simulink library "Prop_demo"  (R2025b)
settings: Solver=VariableStepAuto  StartTime=0.0  StopTime=10.0  RelTol=1e-3
undefined symbols (not defined in the file): cfd2d_ja, cfd2d_jl, cfd2d_kQ, cfd2d_kT, cfd2d_P1_CEF_X, cfd2d_P1_CEF_Y, cfd2d_P1_CEF_Z, cfd2d_P1_CEM_X, cfd2d_P1_CEM_Y, cfd2d_P1_CEM_Z, cfd2d_P5_CEF_X, cfd2d_P5_CEF_Y, cfd2d_P5_CEF_Z, cfd2d_P5_CEM_X, cfd2d_P5_CEM_Y, cfd2d_P5_CEM_Z, cfd3d_ja, cfd3d_jl, cfd3d_P2_CEF_X, cfd3d_P2_CEF_Y, cfd3d_P2_CEF_Z, cfd3d_P2_CEM_X, cfd3d_P2_CEM_Y, cfd3d_P2_CEM_Z, cfd3d_P6_CEF_X, cfd3d_P6_CEF_Y, cfd3d_P6_CEF_Z, cfd3d_P6_CEM_X, cfd3d_P6_CEM_Y, cfd3d_P6_CEM_Z, cfd3d_pitch, CoefBus, DF3000_V2_Prop, magnitude, Prop1, Prop2
libraries: simulink_extras x22, matrix_library x12, sharedtransform x12, simulink x6, DF3000_V2_Common x4
(part 1 of 4)
settings Model: Creator=someone  LastModifiedBy=someone

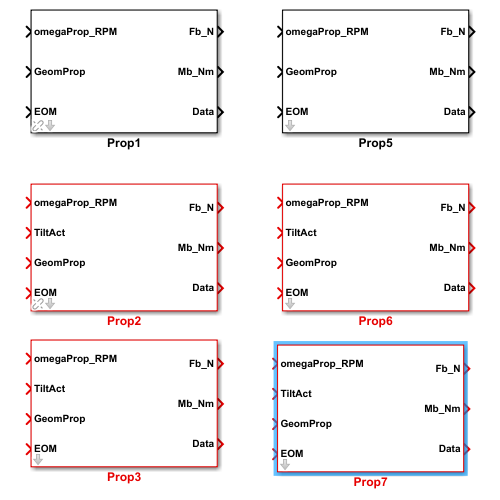
[thumbnail: Simulink's stored preview of the top-level diagram]
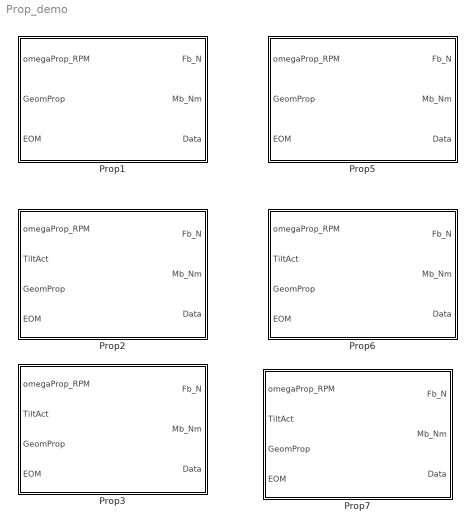
== system Prop_demo ==
  Prop1 : Subsystem  AncestorBlock=DF3000_V2_Prop/Prop1  mask{propAbs=1}
      mask prompts: propAbs "Prop Index"
      mask DialogControl ParameterGroupVar Prompt: 参数
  Prop2 : Subsystem  AncestorBlock=DF3000_V2_Prop/Prop2  mask{propAbs=2, ArmDirSelected=on}
      mask prompts: propAbs "Prop Index"; ArmDirSelected "Positive Installed (Front Prop)"
      mask DialogControl ParameterGroupVar Prompt: 参数
  Prop3 : Subsystem  mask{propAbs=2, ArmDirSelected=on}
      mask prompts: propAbs "Prop Index"; ArmDirSelected "Positive Installed (Front Prop)"
      mask DialogControl ParameterGroupVar Prompt: 参数
  Prop5 : Subsystem  mask{propAbs=5}
      mask prompts: propAbs "Prop Index"
      mask DialogControl ParameterGroupVar Prompt: 参数
  Prop6 : Subsystem  mask{propAbs=6, ArmDirSelected=on}
      mask prompts: propAbs "Prop Index"; ArmDirSelected "Positive Installed (Front Prop)"
      mask DialogControl ParameterGroupVar Prompt: 参数
  Prop7 : Subsystem  mask{propAbs=6, ArmDirSelected=on}
      mask prompts: propAbs "Prop Index"; ArmDirSelected "Positive Installed (Front Prop)"
      mask DialogControl ParameterGroupVar Prompt: 参数

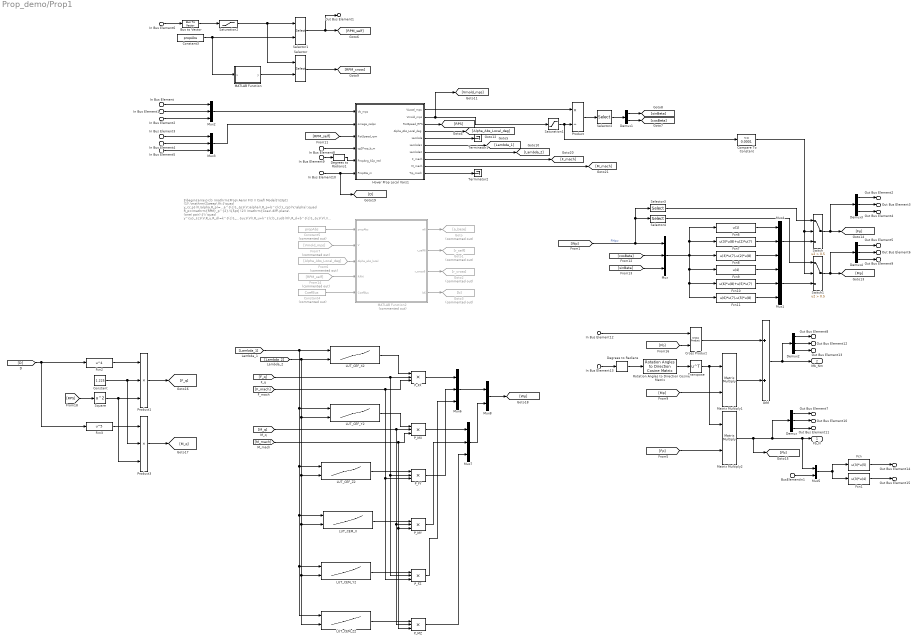
== system Prop_demo/Prop1 ==
  note: $\begin{array}{l} \mathrm{Prop\ Aero\ Fit\ /\ Coef\ Model}\\[3pt] (1)\ \mathrm{Sweep\ fit:}\quad y_{c,p}(V,\alpha,R_p)=a^{(c)}_{p}(V,\alpha)\,R_p+b^{(c)}_{p}(V,\alpha),\quad R_p=\mathrm{RPM}_p^{2}.\\[5pt] (2)\ \mathrm{Coax\ diff\ plane\ (one\ pair):}\\ \quad y^{u}_{c}(V,R_u,R_d)=k^{(c)}_{uu}(V)\,R_u+k^{(c)}_{ud}(V)\,R_d+b^{(c)}_{u}(V),\\ \quad y^{d}_{c}(V,R_u,R_d)=k^{(c)}_{du}(V)\,R_u+k^{(c)}_{dd}(V)\,R_d+b^{(c)}_{d}(V).\\[5pt] (3)\ \mathrm{Ratio\ (split\ of\ slope):}\quad s^{(c)}_{u}=k^{(c)}_{uu}+k^{(c)}_{ud},\quad s^{(c)}_{d}=k^{(c)}_{dd}+k^{(c)}_{du},\\ \quad r^{(c)}_{uu}=\frac{k^{(c)}_{uu}}{s^{(c)}_{u}},\quad r^{(c)}_{ud}=\frac{k^{(c)}_{ud}}{s^{(c)}_{u}},\quad r^{(c)}_{dd}=\frac{k^{(c)}_{dd}}{s^{(c)}_{d}},\quad r^{(c)}_{du}=\frac{k^{(c)}_{du}}{s^{(c)}_{d}}.\\[5pt] (4)\ \mathrm{Coax\ weight:}\quad s=(\cos(\alpha))^{p},\quad p=\mathrm{coaxAlphaPow}.\\ \quad \mathrm{upper:}\quad a^{(c)}_{\mathrm{self}}=s\,r^{(c)}_{uu}\,a^{(c)}_{p},\quad a^{(c)}_{\mathrm{cross}}=s\,r^{(c)}_{ud}\,a^{(c)}_{p},\\ \quad \mathrm{lower:}\quad a^{(c)}_{\mathrm{self}}=s\,r^{(c)}_{dd}\,a^{(c)}_{p},\quad a^{(c)}_{\mathrm{cross}}=s\,r^{(c)}_{du}\,a^{(c)}_{p}.\\[5pt] (5)\ \mathrm{Final\ prediction:}\quad \hat y_{c,p}=a^{(c)}_{\mathrm{self}}\,R_p+a^{(c)}_{\mathrm{cross}}\,R_{m(p)}+b^{(c)}_{p}(V,\alpha). \end{array}$
  In Bus Element6 : Inport  PortName=omegaProp_RPM
      settings: AttributesFormatString=%<OutDataTypeStr>\nDimensions: %<PortDimensions>
  In Bus Element12 : Inport  Port=2  PortName=GeomProp  Element=cg2Prop_b_m
      settings: AttributesFormatString=%<OutDataTypeStr>\nDimensions: %<PortDimensions>
  In Bus Element8 : Inport  Port=2  PortName=GeomProp  Element=cg2Prop_b_m
      settings: AttributesFormatString=%<OutDataTypeStr>\nDimensions: %<PortDimensions>
  In Bus Element13 : Inport  Port=2  PortName=GeomProp  Element=PropAng_b2p_deg
      settings: AttributesFormatString=%<OutDataTypeStr>\nDimensions: %<PortDimensions>
  In Bus Element9 : Inport  Port=2  PortName=GeomProp  Element=PropAng_b2p_deg
      settings: AttributesFormatString=%<OutDataTypeStr>\nDimensions: %<PortDimensions>
  In Bus Element10 : Inport  Port=2  PortName=GeomProp  Element=PropDia_m
      settings: AttributesFormatString=%<OutDataTypeStr>\nDimensions: %<PortDimensions>
  BusElementIn1 : Inport  Port=2  PortName=GeomProp  Element=root2Prop_b_m
  In Bus Element : Inport  Port=3  PortName=EOM  Element=VB_mps.Ub_mps
      settings: AttributesFormatString=%<OutDataTypeStr>\nDimensions: %<PortDimensions>
  In Bus Element1 : Inport  Port=3  PortName=EOM  Element=VB_mps.Vb_mps
      settings: AttributesFormatString=%<OutDataTypeStr>\nDimensions: %<PortDimensions>
  In Bus Element2 : Inport  Port=3  PortName=EOM  Element=VB_mps.Wb_mps
      settings: AttributesFormatString=%<OutDataTypeStr>\nDimensions: %<PortDimensions>
  In Bus Element3 : Inport  Port=3  PortName=EOM  Element=Rates_radps.P_radps
      settings: AttributesFormatString=%<OutDataTypeStr>\nDimensions: %<PortDimensions>
  In Bus Element4 : Inport  Port=3  PortName=EOM  Element=Rates_radps.Q_radps
      settings: AttributesFormatString=%<OutDataTypeStr>\nDimensions: %<PortDimensions>
  In Bus Element5 : Inport  Port=3  PortName=EOM  Element=Rates_radps.R_radps
      settings: AttributesFormatString=%<OutDataTypeStr>\nDimensions: %<PortDimensions>
  Add : Sum
  Bus to Vector : BusToVector
  Compare To Constant : simulink/Logic and Bit Operations/Compare To Constant  relop=<=  const=0.0001  OutDataTypeStr=boolean
  Constant : Constant  Value=1.225
  Constant3 : Constant  Value=propAbs
  Constant4 : Constant  Commented=on  Value=CoefBus  OutDataTypeStr=Bus: CoefBusObj
  Constant5 : Constant  Commented=on  Value=propAbs
  Cross Product : matrix_library/Cross Product
  Degrees to Radians : simulink_extras/Transformations/Degrees to Radians
  Degrees to Radians1 : simulink_extras/Transformations/Degrees to Radians
  Demux{,2..4} (4 alike) : Demux  Outputs=3
  Demux1 : Demux  Outputs=2
  Fcn : Fcn  Expr=u(3)*u(5)
  Fcn1 : Fcn  Expr=u(3)*u(4)
  Fcn10 : Fcn  Expr=u(6)*u(8)+u(5)*u(7)
  Fcn11 : Fcn  Expr=u(6)*u(7)-u(5)*u(8)
  Fcn2 : Fcn  Expr=u^4
  Fcn3 : Fcn  Expr=u^5
  Fcn6 : Fcn  Expr=u(1)
  Fcn7 : Fcn  Expr=u(3)*u(8)+u(2)*u(7)
  Fcn8 : Fcn  Expr=u(3)*u(7)-u(2)*u(8)
  Fcn9 : Fcn  Expr=u(4)
  From14 : From  Commented=on  GotoTag=RPM_self
  From6 : From  Commented=on  GotoTag=Alpha_Abs_Local_deg
  From7 : From  Commented=on  GotoTag=Vmold_mps
  Goto : Goto  Commented=on  GotoTag=a_base
  Goto1 : Goto  Commented=on  GotoTag=r_self
  Goto2 : Goto  Commented=on  GotoTag=r_cross
  Goto3 : Goto  Commented=on  GotoTag=b
  Hover Prop Local Vars1 : Subsystem  AncestorBlock=DF3000_V2_Common/Hover Prop Local Vars1
  LUT_CEF_X2 : Lookup_n-D  BreakpointsForDimension1=cfd2d_ja  BreakpointsForDimension2=cfd2d_jl  BreakpointsForDimension3=[5, 7]  Table=cfd2d_P1_CEF_X  ExtrapMethod=Clip  UseLastTableValue=on  InternalRulePriority=Speed  RndMeth=Simplest
      settings: InputPortMap=u0,u1
  LUT_CEF_Y2 : Lookup_n-D  BreakpointsForDimension1=cfd2d_ja  BreakpointsForDimension2=cfd2d_jl  BreakpointsForDimension3=[5, 7]  Table=cfd2d_P1_CEM_X  ExtrapMethod=Clip  UseLastTableValue=on  InternalRulePriority=Speed  RndMeth=Simplest
      settings: InputPortMap=u0,u1
  LUT_CEF_Z2 : Lookup_n-D  BreakpointsForDimension1=cfd2d_ja  BreakpointsForDimension2=cfd2d_jl  BreakpointsForDimension3=[5, 7]  Table=cfd2d_P1_CEF_Y  ExtrapMethod=Clip  UseLastTableValue=on  InternalRulePriority=Speed  RndMeth=Simplest
      settings: InputPortMap=u0,u1
  LUT_CEM_X : Lookup_n-D  BreakpointsForDimension1=cfd2d_ja  BreakpointsForDimension2=cfd2d_jl  BreakpointsForDimension3=[5, 7]  Table=cfd2d_P1_CEM_Y  ExtrapMethod=Clip  UseLastTableValue=on  InternalRulePriority=Speed  RndMeth=Simplest
      settings: InputPortMap=u0,u1
  LUT_CEM_Y2 : Lookup_n-D  BreakpointsForDimension1=cfd2d_ja  BreakpointsForDimension2=cfd2d_jl  BreakpointsForDimension3=[5, 7]  Table=cfd2d_P1_CEF_Z  ExtrapMethod=Clip  UseLastTableValue=on  InternalRulePriority=Speed  RndMeth=Simplest
      settings: InputPortMap=u0,u1
  LUT_CEM_Z2 : Lookup_n-D  BreakpointsForDimension1=cfd2d_ja  BreakpointsForDimension2=cfd2d_jl  BreakpointsForDimension3=[5, 7]  Table=cfd2d_P1_CEM_Z  ExtrapMethod=Clip  UseLastTableValue=on  InternalRulePriority=Speed  RndMeth=Simplest
      settings: InputPortMap=u0,u1
  MATLAB Function : MATLAB Function  TreatAsAtomicUnit=on
  MATLAB Function2 : MATLAB Function  Commented=on  TreatAsAtomicUnit=on
  Matrix Multiply1 : Product  Multiplication=Matrix(*)
  Matrix Multiply2 : Product  Multiplication=Matrix(*)
  Mux{,1..4,6..7} (7 alike) : Mux  Inputs=3
  Mux5 : Mux  Inputs=2
  Mux8 : Mux  Inputs=2
  P_FX : Product  Inputs=***
  P_FY : Product  Inputs=***
  P_FZ : Product  Inputs=***
  P_MX : Product  Inputs=***
  P_MY : Product  Inputs=***
  P_MZ : Product  Inputs=***
  Product : Product  Inputs=*/
  Product1 : Product  Inputs=3
  Product3 : Product  Inputs=3
  Rotation Angles to Direction Cosine Matrix : sharedtransform/Rotation Angles to Direction Cosine Matrix  rotationOrder=XYZ  aMode=aMode
  Saturation1 : Saturate  UpperLimit=inf  LowerLimit=0.0001
  Saturation2 : Saturate  UpperLimit=1500  LowerLimit=0
      settings: AttributesFormatString=min: %<LowerLimit>\nmax: %<UpperLimit>
  Selector : Selector  InputPortWidth=8  IndexOptions=Index vector (port)  Indices=[1 3]  OutputSizes=1
  Selector1 : Selector  InputPortWidth=8  IndexOptions=Index vector (port)  Indices=[1 3]  OutputSizes=1
  Selector2 : Selector  InputPortWidth=3  IndexOptions=Index vector (dialog)  Indices=[2 3]  OutputSizes=1
  Selector3 : Selector  InputPortWidth=6  IndexOptions=Index vector (dialog)  Indices=[1 2 3]  OutputSizes=1
  Selector4 : Selector  InputPortWidth=6  IndexOptions=Index vector (dialog)  Indices=[4 5 6]  OutputSizes=1
  Square : Math  Operator=square
  Switch : Switch  Criteria=u2 > Threshold  Threshold=0.5  SaturateOnIntegerOverflow=off  InputSameDT=off
  Switch1 : Switch  Criteria=u2 > Threshold  Threshold=0.5  SaturateOnIntegerOverflow=off  InputSameDT=off
  Terminator1 : Terminator
  Terminator2 : Terminator
  Transpose : Math  Operator=transpose
  Fb_N : Outport  PortDimensions=3
  Mb_Nm : Outport  Port=2  PortDimensions=3
  Out Bus Element7 : Outport  Port=3  PortName=Data  Element=Fx_Prop
  Out Bus Element10 : Outport  Port=3  PortName=Data  Element=Fy_Prop
  Out Bus Element11 : Outport  Port=3  PortName=Data  Element=Fz_Prop
  Out Bus Element8 : Outport  Port=3  PortName=Data  Element=Mx_Prop
  Out Bus Element12 : Outport  Port=3  PortName=Data  Element=My_Prop
  Out Bus Element13 : Outport  Port=3  PortName=Data  Element=Mz_Prop
  Out Bus Element1 : Outport  Port=3  PortName=Data  Element=RPM
  Out Bus Element2 : Outport  Port=3  PortName=Data  Element=Fx_Local
  Out Bus Element3 : Outport  Port=3  PortName=Data  Element=Fy_Local
  Out Bus Element4 : Outport  Port=3  PortName=Data  Element=Fz_Local
  Out Bus Element5 : Outport  Port=3  PortName=Data  Element=Mx_Local
  Out Bus Element6 : Outport  Port=3  PortName=Data  Element=My_Local
  Out Bus Element9 : Outport  Port=3  PortName=Data  Element=Mz_Local
  Out Bus Element14 : Outport  Port=3  PortName=Data  Element=BMbx_Prop
  Out Bus Element15 : Outport  Port=3  PortName=Data  Element=BMby_Prop
  wires:
  Fcn1/1 -> Out Bus Element15/1
  Fcn/1 -> Out Bus Element14/1
  Mux5/1 -> Fcn/1, Fcn1/1
  BusElementIn1/1 -> Mux5/2
  From14/1 -> MATLAB Function2/4(RPM)
  Demux4/2 -> Out Bus Element6/1
  Demux4/1 -> Out Bus Element5/1
  Demux4/3 -> Out Bus Element9/1
  Demux3/3 -> Out Bus Element4/1
  Demux3/1 -> Out Bus Element2/1
  Demux3/2 -> Out Bus Element3/1
  Selector3/1 -> Switch/1
  Switch/1 -> [Fp], Demux3/1
  Selector4/1 -> Switch1/1
  Mux4/1 -> Switch/3
  Saturation1/1 -> Product/2, Compare To Constant/1
  Compare To Constant/1 -> Switch/2, Switch1/2
  Mux1/1 -> Switch1/3
  Switch1/1 -> [Mp], Demux4/1
  Demux1/1 -> [sinBeta]
  Demux1/2 -> [cosBeta]
  Selector/1 -> [RPM_cross]
  MATLAB Function/1(y) -> Selector/2
  Constant3/1 -> Selector1/2, MATLAB Function/1(u)
  In Bus Element6/1 -> Bus to Vector/1
  Bus to Vector/1 -> Saturation2/1
  Saturation2/1 -> Selector/1, Selector1/1
  MATLAB Function2/1(a6) -> Goto/1
  Rotation Angles to Direction Cosine Matrix/1 -> Transpose/1
  In Bus Element12/1 -> Cross Product/1
  Cross Product/1 -> Add/1
  In Bus Element13/1 -> Degrees to Radians/1
  Degrees to Radians/1 -> Rotation Angles to Direction Cosine Matrix/1
  Matrix Multiply1/1 -> Add/2
  [Mp] -> Matrix Multiply1/2
  Transpose/1 -> Matrix Multiply2/1, Matrix Multiply1/1
  Selector1/1 -> [RPM_self], Out Bus Element1/1
  In Bus Element8/1 -> Hover Prop Local Vars1/4(cg2Prop_b_m)
  In Bus Element9/1 -> Degrees to Radians1/1
  In Bus Element/1 -> Mux2/1
  In Bus Element5/1 -> Mux3/3
  In Bus Element4/1 -> Mux3/2
  In Bus Element3/1 -> Mux3/1
  In Bus Element2/1 -> Mux2/3
  In Bus Element10/1 -> [D], Hover Prop Local Vars1/6(PropDia_m)
  Mux3/1 -> Hover Prop Local Vars1/2(omega_radps)
  Mux2/1 -> Hover Prop Local Vars1/1(Vb_mps)
  In Bus Element1/1 -> Mux2/2
  [RPM_self] -> Hover Prop Local Vars1/3(RotSpeed_rpm)
  Hover Prop Local Vars1/1(VLocal_mps) -> Product/1
  Hover Prop Local Vars1/2(Vmold_mps) -> [Vmold_mps], Saturation1/1
  Product/1 -> Selector2/1
  Selector2/1 -> Demux1/1
  Hover Prop Local Vars1/3(RotSpeed_RPS) -> [RPS]
  Hover Prop Local Vars1/5(Lambda) -> Terminator1/1
  Constant4/1 -> MATLAB Function2/5(CoefBus)
  Constant5/1 -> MATLAB Function2/1(propAbs)
  MATLAB Function2/4(b6) -> Goto3/1
  MATLAB Function2/3(r_cross6) -> Goto2/1
  MATLAB Function2/2(r_self6) -> Goto1/1
  Hover Prop Local Vars1/4(Alpha_Abs_Local_deg) -> [Alpha_Abs_Local_deg]
  From6/1 -> MATLAB Function2/3(Alpha_abs_local)
  From7/1 -> MATLAB Function2/2(V)
  [cosBeta] -> Mux/2
  [sinBeta] -> Mux/3
  Mux/1 -> Fcn7/1, Fcn6/1, Fcn10/1, Fcn11/1, Fcn9/1, Fcn8/1
  Fcn9/1 -> Mux1/1
  Fcn10/1 -> Mux1/2
  Fcn11/1 -> Mux1/3
  Fcn6/1 -> Mux4/1
  Fcn7/1 -> Mux4/2
  Fcn8/1 -> Mux4/3
  [Fp] -> Matrix Multiply2/2
  Matrix Multiply2/1 -> Demux/1, Fb_N/1, Mux5/1, [Fb]
  [Fb] -> Cross Product/2
  [Wp] -> Mux/1, Selector3/1, Selector4/1  "FMpw"
  Demux/1 -> Out Bus Element7/1
  Demux/2 -> Out Bus Element10/1
  Demux/3 -> Out Bus Element11/1
  Demux2/3 -> Out Bus Element13/1
  Demux2/2 -> Out Bus Element12/1
  Demux2/1 -> Out Bus Element8/1
  Add/1 -> Mb_Nm/1, Demux2/1
  Degrees to Radians1/1 -> Hover Prop Local Vars1/5(PropAng_b2p_rad)
  [RPS] -> Square/1
  Square/1 -> Product3/3, Product1/3
  Product3/1 -> [M_q]
  Constant/1 -> Product3/2, Product1/2
  Product1/1 -> [F_q]
  Fcn2/1 -> Product1/1
  Fcn3/1 -> Product3/1
  LUT_CEM_Z2/1 -> P_MZ/1
  LUT_CEF_Z2/1 -> P_FY/1
  [M_q] -> P_MZ/2, P_MY/2, P_MX/2
  [M_mach] -> P_MZ/3, P_MY/3, P_MX/3
  LUT_CEF_X2/1 -> P_FX/1
  LUT_CEM_Y2/1 -> P_FZ/1
  [Lambda_1] -> LUT_CEM_Z2/1, LUT_CEM_Y2/1, LUT_CEM_X/1, LUT_CEF_Z2/1, LUT_CEF_Y2/1, LUT_CEF_X2/1
  P_FX/1 -> Mux6/1
  [Lambda_2] -> LUT_CEM_Z2/2, LUT_CEM_Y2/2, LUT_CEM_X/2, LUT_CEF_Z2/2, LUT_CEF_Y2/2, LUT_CEF_X2/2
  LUT_CEM_X/1 -> P_MY/1
  P_MX/1 -> Mux7/1
  LUT_CEF_Y2/1 -> P_MX/1
  [F_mach] -> P_FZ/3, P_FY/3, P_FX/3
  [F_q] -> P_FZ/2, P_FY/2, P_FX/2
  Hover Prop Local Vars1/6(Lambda1) -> [Lambda_1]
  Hover Prop Local Vars1/7(Lambda2) -> [Lambda_2]
  Hover Prop Local Vars1/8(F_mach) -> [F_mach]
  Hover Prop Local Vars1/9(M_mach) -> [M_mach]
  Hover Prop Local Vars1/10(Tip_mach) -> Terminator2/1
  P_FY/1 -> Mux6/2
  P_FZ/1 -> Mux6/3
  P_MY/1 -> Mux7/2
  P_MZ/1 -> Mux7/3
  Mux6/1 -> Mux8/1
  Mux7/1 -> Mux8/2
  Mux8/1 -> [Wp]
  [D] -> Fcn3/1, Fcn2/1

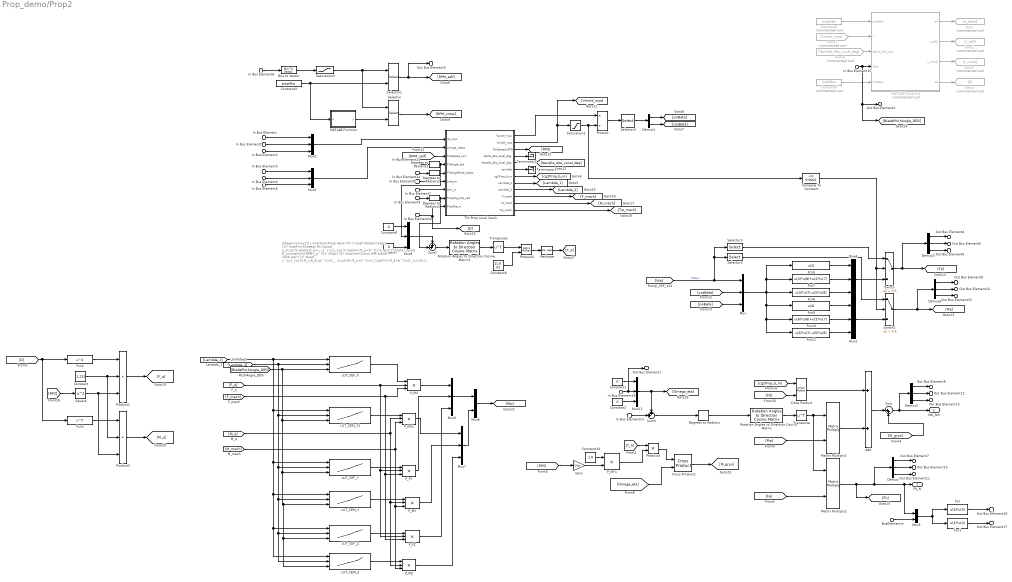
== system Prop_demo/Prop2 ==
  note: $\begin{array}{l} \mathrm{Prop\ Aero\ Fit\ /\ Coef\ Model}\\[3pt] (1)\ \mathrm{Sweep\ fit:}\quad y_{c,p}(V,\alpha,R_p)=a^{(c)}_{p}(V,\alpha)\,R_p+b^{(c)}_{p}(V,\alpha),\quad R_p=\mathrm{RPM}_p^{2}.\\[5pt] (2)\ \mathrm{Coax\ diff\ plane\ (one\ pair):}\\ \quad y^{u}_{c}(V,R_u,R_d)=k^{(c)}_{uu}(V)\,R_u+k^{(c)}_{ud}(V)\,R_d+b^{(c)}_{u}(V),\\ \quad y^{d}_{c}(V,R_u,R_d)=k^{(c)}_{du}(V)\,R_u+k^{(c)}_{dd}(V)\,R_d+b^{(c)}_{d}(V).\\[5pt] (3)\ \mathrm{Ratio\ (split\ of\ slope):}\quad s^{(c)}_{u}=k^{(c)}_{uu}+k^{(c)}_{ud},\quad s^{(c)}_{d}=k^{(c)}_{dd}+k^{(c)}_{du},\\ \quad r^{(c)}_{uu}=\frac{k^{(c)}_{uu}}{s^{(c)}_{u}},\quad r^{(c)}_{ud}=\frac{k^{(c)}_{ud}}{s^{(c)}_{u}},\quad r^{(c)}_{dd}=\frac{k^{(c)}_{dd}}{s^{(c)}_{d}},\quad r^{(c)}_{du}=\frac{k^{(c)}_{du}}{s^{(c)}_{d}}.\\[5pt] (4)\ \mathrm{Coax\ weight:}\quad s=(\cos(\alpha))^{p},\quad p=\mathrm{coaxAlphaPow}.\\ \quad \mathrm{upper:}\quad a^{(c)}_{\mathrm{self}}=s\,r^{(c)}_{uu}\,a^{(c)}_{p},\quad a^{(c)}_{\mathrm{cross}}=s\,r^{(c)}_{ud}\,a^{(c)}_{p},\\ \quad \mathrm{lower:}\quad a^{(c)}_{\mathrm{self}}=s\,r^{(c)}_{dd}\,a^{(c)}_{p},\quad a^{(c)}_{\mathrm{cross}}=s\,r^{(c)}_{du}\,a^{(c)}_{p}.\\[5pt] (5)\ \mathrm{Final\ prediction:}\quad \hat y_{c,p}=a^{(c)}_{\mathrm{self}}\,R_p+a^{(c)}_{\mathrm{cross}}\,R_{m(p)}+b^{(c)}_{p}(V,\alpha). \end{array}$
  In Bus Element6 : Inport  PortName=omegaProp_RPM
      settings: AttributesFormatString=%<OutDataTypeStr>\nDimensions: %<PortDimensions>
  In Bus Element14 : Inport  Port=2  PortName=TiltAct  Element=TiltAngleRate_dps
  In Bus Element15 : Inport  Port=2  PortName=TiltAct  Element=BladePitchAngle_DEG
  In Bus Element11 : Inport  Port=2  PortName=TiltAct  Element=TiltAngle_DEG
  In Bus Element16 : Inport  Port=2  PortName=TiltAct  Element=TiltAngle_DEG
  In Bus Element13 : Inport  Port=3  PortName=GeomProp  Element=PropAng_b2p_deg
      settings: AttributesFormatString=%<OutDataTypeStr>\nDimensions: %<PortDimensions>
  In Bus Element9 : Inport  Port=3  PortName=GeomProp  Element=PropAng_b2p_deg
      settings: AttributesFormatString=%<OutDataTypeStr>\nDimensions: %<PortDimensions>
  In Bus Element10 : Inport  Port=3  PortName=GeomProp  Element=PropDia_m
      settings: AttributesFormatString=%<OutDataTypeStr>\nDimensions: %<PortDimensions>
  In Bus Element8 : Inport  Port=3  PortName=GeomProp  Element=cg2PropHinge_b_m
      settings: AttributesFormatString=%<OutDataTypeStr>\nDimensions: %<PortDimensions>
  BusElementIn : Inport  Port=3  PortName=GeomProp  Element=cg2PropHinge_b_m
  In Bus Element7 : Inport  Port=3  PortName=GeomProp  Element=TiltArm_m
      settings: AttributesFormatString=%<OutDataTypeStr>\nDimensions: %<PortDimensions>
  In Bus Element : Inport  Port=4  PortName=EOM  Element=VB_mps.Ub_mps
      settings: AttributesFormatString=%<OutDataTypeStr>\nDimensions: %<PortDimensions>
  In Bus Element1 : Inport  Port=4  PortName=EOM  Element=VB_mps.Vb_mps
      settings: AttributesFormatString=%<OutDataTypeStr>\nDimensions: %<PortDimensions>
  In Bus Element2 : Inport  Port=4  PortName=EOM  Element=VB_mps.Wb_mps
      settings: AttributesFormatString=%<OutDataTypeStr>\nDimensions: %<PortDimensions>
  In Bus Element3 : Inport  Port=4  PortName=EOM  Element=Rates_radps.P_radps
      settings: AttributesFormatString=%<OutDataTypeStr>\nDimensions: %<PortDimensions>
  In Bus Element4 : Inport  Port=4  PortName=EOM  Element=Rates_radps.Q_radps
      settings: AttributesFormatString=%<OutDataTypeStr>\nDimensions: %<PortDimensions>
  In Bus Element5 : Inport  Port=4  PortName=EOM  Element=Rates_radps.R_radps
      settings: AttributesFormatString=%<OutDataTypeStr>\nDimensions: %<PortDimensions>
  Add : Sum
  Bus to Vector : BusToVector
  Compare To Constant : simulink/Logic and Bit Operations/Compare To Constant  relop=<=  const=0.0001  OutDataTypeStr=boolean
  Constant : Constant  Value=1.225
  Constant{1..2,6..7} (4 alike) : Constant  Value=0
  Constant10 : Constant  Value=1.0
  Constant3 : Constant  Value=propAbs
  Constant4 : Constant  Commented=on  Value=CoefBus  OutDataTypeStr=Bus: CoefBusObj
  Constant5 : Constant  Commented=on  Value=propAbs
  Constant8 : Constant  Value=[1 0 0]
  Cross Product : matrix_library/Cross Product
  Cross Product2 : matrix_library/Cross Product
  Degrees to Radians{,1..3} (4 alike) : simulink_extras/Transformations/Degrees to Radians
  Demux{,2..4} (4 alike) : Demux  Outputs=3
  Demux1 : Demux  Outputs=2
  Fcn : Fcn  Expr=u(3)*u(5)
  Fcn1 : Fcn  Expr=u(3)*u(4)
  Fcn10 : Fcn  Expr=u(6)*u(8)+u(5)*u(7)
  Fcn11 : Fcn  Expr=u(6)*u(7)-u(5)*u(8)
  Fcn2 : Fcn  Expr=u^4
  Fcn3 : Fcn  Expr=u^5
  Fcn6 : Fcn  Expr=u(1)
  Fcn7 : Fcn  Expr=u(3)*u(8)+u(2)*u(7)
  Fcn8 : Fcn  Expr=u(3)*u(7)-u(2)*u(8)
  Fcn9 : Fcn  Expr=u(4)
  From6 : From  Commented=on  GotoTag=Nacelle_Abs_Local_deg
  From7 : From  Commented=on  GotoTag=Vmold_mps
  Gain : Gain  Gain=-2*pi
  Goto : Goto  Commented=on  GotoTag=a_base
  Goto1 : Goto  Commented=on  GotoTag=r_self
  Goto2 : Goto  Commented=on  GotoTag=r_cross
  Goto3 : Goto  Commented=on  GotoTag=b
  LUT_CEF_X : Lookup_n-D  NumberOfTableDimensions=3  BreakpointsForDimension1=cfd3d_ja  BreakpointsForDimension2=cfd3d_jl  BreakpointsForDimension3=cfd3d_pitch  Table=cfd3d_P2_CEF_X  ExtrapMethod=Clip  UseLastTableValue=on  InternalRulePriority=Speed  RndMeth=Simplest
      settings: InputPortMap=u0,u1,u2
  LUT_CEF_Y : Lookup_n-D  NumberOfTableDimensions=3  BreakpointsForDimension1=cfd3d_ja  BreakpointsForDimension2=cfd3d_jl  BreakpointsForDimension3=cfd3d_pitch  Table=cfd3d_P2_CEF_Y  ExtrapMethod=Clip  UseLastTableValue=on  InternalRulePriority=Speed  RndMeth=Simplest
      settings: InputPortMap=u0,u1,u2
  LUT_CEF_Z : Lookup_n-D  NumberOfTableDimensions=3  BreakpointsForDimension1=cfd3d_ja  BreakpointsForDimension2=cfd3d_jl  BreakpointsForDimension3=cfd3d_pitch  Table=cfd3d_P2_CEF_Z  ExtrapMethod=Clip  UseLastTableValue=on  InternalRulePriority=Speed  RndMeth=Simplest
      settings: InputPortMap=u0,u1,u2
  LUT_CEM_X1 : Lookup_n-D  NumberOfTableDimensions=3  BreakpointsForDimension1=cfd3d_ja  BreakpointsForDimension2=cfd3d_jl  BreakpointsForDimension3=cfd3d_pitch  Table=cfd3d_P2_CEM_X  ExtrapMethod=Clip  UseLastTableValue=on  InternalRulePriority=Speed  RndMeth=Simplest
      settings: InputPortMap=u0,u1,u2
  LUT_CEM_Y : Lookup_n-D  NumberOfTableDimensions=3  BreakpointsForDimension1=cfd3d_ja  BreakpointsForDimension2=cfd3d_jl  BreakpointsForDimension3=cfd3d_pitch  Table=cfd3d_P2_CEM_Y  ExtrapMethod=Clip  UseLastTableValue=on  InternalRulePriority=Speed  RndMeth=Simplest
      settings: InputPortMap=u0,u1,u2
  LUT_CEM_Z : Lookup_n-D  NumberOfTableDimensions=3  BreakpointsForDimension1=cfd3d_ja  BreakpointsForDimension2=cfd3d_jl  BreakpointsForDimension3=cfd3d_pitch  Table=cfd3d_P2_CEM_Z  ExtrapMethod=Clip  UseLastTableValue=on  InternalRulePriority=Speed  RndMeth=Simplest
      settings: InputPortMap=u0,u1,u2
  MATLAB Function : MATLAB Function  TreatAsAtomicUnit=on
  MATLAB Function2 : MATLAB Function  Commented=on  TreatAsAtomicUnit=on
  Matrix Multiply1 : Product  Multiplication=Matrix(*)
  Matrix Multiply2 : Product  Multiplication=Matrix(*)
  Mux{,1..4,6..7,9,11} (9 alike) : Mux  Inputs=3
  Mux5 : Mux  Inputs=2
  Mux8 : Mux  Inputs=2
  P_FY : Product  Inputs=***
  P_FZ : Product  Inputs=***
  P_MX : Product  Inputs=***
  P_MX1 : Product  Inputs=***
  P_MY : Product  Inputs=***
  P_MY1 : Product  Inputs=**
  P_MZ : Product  Inputs=***
  Product : Product  Inputs=*/
  Product1 : Product  Inputs=3
  Product2 : Product  Multiplication=Matrix(*)
  Product3 : Product  Inputs=3
  Product4 : Product
  Reshape : Reshape
  Rotation Angles to Direction Cosine Matrix : sharedtransform/Rotation Angles to Direction Cosine Matrix  rotationOrder=XYZ  aMode=aMode
  Rotation Angles to Direction Cosine Matrix1 : sharedtransform/Rotation Angles to Direction Cosine Matrix  rotationOrder=XYZ  aMode=aMode
  Saturation1 : Saturate  UpperLimit=inf  LowerLimit=0.0001
  Saturation2 : Saturate  UpperLimit=1500  LowerLimit=0
      settings: AttributesFormatString=min: %<LowerLimit>\nmax: %<UpperLimit>
  Selector : Selector  InputPortWidth=8  IndexOptions=Index vector (port)  Indices=[1 3]  OutputSizes=1
  Selector1 : Selector  InputPortWidth=8  IndexOptions=Index vector (port)  Indices=[1 3]  OutputSizes=1
  Selector2 : Selector  InputPortWidth=3  IndexOptions=Index vector (dialog)  Indices=[2 3]  OutputSizes=1
  Selector3 : Selector  InputPortWidth=6  IndexOptions=Index vector (dialog)  Indices=[1 2 3]  OutputSizes=1
  Selector4 : Selector  InputPortWidth=6  IndexOptions=Index vector (dialog)  Indices=[4 5 6]  OutputSizes=1
  Square : Math  Operator=square
  Sum : Sum  Inputs=|++
  Sum1 : Sum  Inputs=++|
  Sum5 : Sum  Inputs=++|
  Switch : Switch  Criteria=u2 > Threshold  Threshold=0.5  SaturateOnIntegerOverflow=off  InputSameDT=off
  Switch1 : Switch  Criteria=u2 > Threshold  Threshold=0.5  SaturateOnIntegerOverflow=off  InputSameDT=off
  Terminator1 : Terminator
  Terminator2 : Terminator
  Tilt Prop Local Vars1 : Subsystem  AncestorBlock=DF3000_V2_Common/Tilt Prop Local Vars1
  Transpose : Math  Operator=transpose
  Transpose1 : Math  Operator=transpose
  Fb_N : Outport  PortDimensions=3
  Mb_Nm : Outport  Port=2  PortDimensions=3
  Out Bus Element7 : Outport  Port=3  PortName=Data  Element=Fx_Prop
  Out Bus Element10 : Outport  Port=3  PortName=Data  Element=Fy_Prop
  Out Bus Element11 : Outport  Port=3  PortName=Data  Element=Fz_Prop
  Out Bus Element8 : Outport  Port=3  PortName=Data  Element=Mx_Prop
  Out Bus Element12 : Outport  Port=3  PortName=Data  Element=My_Prop
  Out Bus Element13 : Outport  Port=3  PortName=Data  Element=Mz_Prop
  Out Bus Element1 : Outport  Port=3  PortName=Data  Element=TiltAngle_DEG
  Out Bus Element2 : Outport  Port=3  PortName=Data  Element=BladePitchAngle_DEG
  Out Bus Element3 : Outport  Port=3  PortName=Data  Element=RPM
  Out Bus Element4 : Outport  Port=3  PortName=Data  Element=Fx_Local
  Out Bus Element5 : Outport  Port=3  PortName=Data  Element=Fy_Local
  Out Bus Element6 : Outport  Port=3  PortName=Data  Element=Fz_Local
  Out Bus Element9 : Outport  Port=3  PortName=Data  Element=Mx_Local
  Out Bus Element14 : Outport  Port=3  PortName=Data  Element=My_Local
  Out Bus Element15 : Outport  Port=3  PortName=Data  Element=Mz_Local
  Out Bus Element16 : Outport  Port=3  PortName=Data  Element=BMbx_Prop
  Out Bus Element17 : Outport  Port=3  PortName=Data  Element=BMby_Prop
  wires:
  Fcn1/1 -> Out Bus Element17/1
  BusElementIn/1 -> Mux5/2
  Mux5/1 -> Fcn/1, Fcn1/1
  Fcn/1 -> Out Bus Element16/1
  Matrix Multiply2/1 -> [Fb], Fb_N/1, Mux5/1, Demux/1
  Demux4/2 -> Out Bus Element14/1
  Demux4/1 -> Out Bus Element9/1
  Switch1/1 -> Demux4/1, [Mp]
  Demux4/3 -> Out Bus Element15/1
  Demux3/2 -> Out Bus Element5/1
  Demux3/1 -> Out Bus Element4/1
  Demux3/3 -> Out Bus Element6/1
  Switch/1 -> [Fp], Demux3/1
  Compare To Constant/1 -> Switch/2, Switch1/2
  Selector4/1 -> Switch1/1
  Selector3/1 -> Switch/1
  Saturation1/1 -> Product/2, Compare To Constant/1
  Tilt Prop Local Vars1/7(cg2Prop_b_m) -> [cg2Prop_b_m]
  Tilt Prop Local Vars1/5(Nacelle_Abs_Local_deg) -> [Nacelle_Abs_Local_deg]
  Tilt Prop Local Vars1/4(Alpha_Abs_Local_deg) -> Terminator2/1
  Demux1/2 -> [cosBeta]
  Demux1/1 -> [sinBeta]
  In Bus Element13/1 -> Sum5/2
  In Bus Element16/1 -> Mux11/2, Out Bus Element1/1
  Constant1/1 -> Mux11/1
  Constant2/1 -> Mux11/3
  Mux11/1 -> [Omega_eta], Sum5/1
  Sum/1 -> Demux2/1, Mb_Nm/1
  Demux2/1 -> Out Bus Element8/1
  Demux2/2 -> Out Bus Element12/1
  Demux2/3 -> Out Bus Element13/1
  Demux/3 -> Out Bus Element11/1
  Demux/2 -> Out Bus Element10/1
  Demux/1 -> Out Bus Element7/1
  [Wp] -> Mux/1, Selector3/1, Selector4/1  "FMpw"
  [Fb] -> Cross Product/2
  [Fp] -> Matrix Multiply2/2
  Mux4/1 -> Switch/3
  Fcn8/1 -> Mux4/3
  Fcn7/1 -> Mux4/2
  Fcn6/1 -> Mux4/1
  Mux1/1 -> Switch1/3
  Fcn11/1 -> Mux1/3
  Fcn10/1 -> Mux1/2
  Fcn9/1 -> Mux1/1
  Mux/1 -> Fcn10/1, Fcn11/1, Fcn9/1, Fcn6/1, Fcn7/1, Fcn8/1
  [sinBeta] -> Mux/3
  [cosBeta] -> Mux/2
  From7/1 -> MATLAB Function2/2(V)
  From6/1 -> MATLAB Function2/3(Alpha_abs_local)
  MATLAB Function2/2(r_self6) -> Goto1/1
  MATLAB Function2/3(r_cross6) -> Goto2/1
  MATLAB Function2/4(b6) -> Goto3/1
  Constant5/1 -> MATLAB Function2/1(propAbs)
  Constant4/1 -> MATLAB Function2/5(CoefBus)
  Tilt Prop Local Vars1/6(Lambda) -> Terminator1/1
  Tilt Prop Local Vars1/3(RotSpeed_RPS) -> [RPS]
  Selector2/1 -> Demux1/1
  Product/1 -> Selector2/1
  Tilt Prop Local Vars1/2(Vmold_mps) -> [Vmold_mps], Saturation1/1
  Tilt Prop Local Vars1/1(VLocal_mps) -> Product/1
  [RPM_self] -> Tilt Prop Local Vars1/3(RotSpeed_rpm)
  In Bus Element1/1 -> Mux2/2
  Mux2/1 -> Tilt Prop Local Vars1/1(Vb_mps)
  Mux3/1 -> Tilt Prop Local Vars1/2(omega_radps)
  In Bus Element10/1 -> [D], Tilt Prop Local Vars1/9(PropDia_m)
  In Bus Element2/1 -> Mux2/3
  In Bus Element3/1 -> Mux3/1
  In Bus Element4/1 -> Mux3/2
  In Bus Element5/1 -> Mux3/3
  In Bus Element/1 -> Mux2/1
  In Bus Element9/1 -> Degrees to Radians1/1
  In Bus Element8/1 -> Tilt Prop Local Vars1/6(Lvec_m)
  Selector1/1 -> [RPM_self], Out Bus Element3/1
  Transpose/1 -> Matrix Multiply1/1, Matrix Multiply2/1
  [Mp] -> Matrix Multiply1/2
  Matrix Multiply1/1 -> Add/2
  Degrees to Radians/1 -> Rotation Angles to Direction Cosine Matrix/1
  Sum5/1 -> Degrees to Radians/1
  Cross Product/1 -> Add/1
  [cg2Prop_b_m] -> Cross Product/1
  Rotation Angles to Direction Cosine Matrix/1 -> Transpose/1
  MATLAB Function2/1(a6) -> Goto/1
  Saturation2/1 -> Selector1/1, Selector/1
  Bus to Vector/1 -> Saturation2/1
  In Bus Element6/1 -> Bus to Vector/1
  Constant3/1 -> MATLAB Function/1(u), Selector1/2
  MATLAB Function/1(y) -> Selector/2
  Selector/1 -> [RPM_cross]
  In Bus Element7/1 -> Tilt Prop Local Vars1/7(Arm_m)
  Degrees to Radians2/1 -> Tilt Prop Local Vars1/5(TiltAngleRate_radps)
  In Bus Element14/1 -> Degrees to Radians2/1
  In Bus Element11/1 -> Degrees to Radians3/1
  In Bus Element15/1 -> MATLAB Function2/4(Pitch), [BladePitchAngle_DEG], Out Bus Element2/1
  Tilt Prop Local Vars1/8(Lambda_1) -> [Lambda_1]
  Tilt Prop Local Vars1/9(Lambda_2) -> [Lambda_2]
  Tilt Prop Local Vars1/10(F_mach) -> [F_mach]
  Tilt Prop Local Vars1/11(M_mach) -> [M_mach]
  Tilt Prop Local Vars1/12(Tip_mach) -> [Tip_mach]
  [F_q] -> P_MX/2, P_FZ/2, P_FY/2
  [M_mach] -> P_MX1/3, P_MZ/3, P_MY/3
  LUT_CEF_Y/1 -> P_FY/1
  [F_mach] -> P_MX/3, P_FZ/3, P_FY/3
  LUT_CEM_Z/1 -> P_MZ/1
  LUT_CEM_Y/1 -> P_MY/1
  LUT_CEM_X1/1 -> P_MX1/1
  [M_q] -> P_MZ/2, P_MY/2, P_MX1/2
  [Lambda_2] -> LUT_CEM_Z/2, LUT_CEF_Z/2, LUT_CEM_Y/2, LUT_CEF_Y/2, LUT_CEM_X1/2, LUT_CEF_X/2
  [Lambda_1] -> LUT_CEF_X/1, LUT_CEM_Z/1, LUT_CEF_Z/1, LUT_CEM_Y/1, LUT_CEF_Y/1, LUT_CEM_X1/1
  [BladePitchAngle_DEG] -> LUT_CEM_Z/3, LUT_CEF_Z/3, LUT_CEM_Y/3, LUT_CEF_Y/3, LUT_CEM_X1/3, LUT_CEF_X/3
  LUT_CEF_Z/1 -> P_FZ/1
  LUT_CEF_X/1 -> P_MX/1
  P_MX/1 -> Mux6/1
  P_MY/1 -> Mux7/2
  P_MZ/1 -> Mux7/3
  P_FY/1 -> Mux6/2
  Mux6/1 -> Mux8/1
  Mux7/1 -> Mux8/2
  Mux8/1 -> [Wp]
  P_FZ/1 -> Mux6/3
  P_MX1/1 -> Mux7/1
  Fcn2/1 -> Product1/1
  [D] -> Fcn3/1, Fcn2/1
  Fcn3/1 -> Product3/1
  Product1/1 -> [F_q]
  Product3/1 -> [M_q]
  Square/1 -> Product3/3, Product1/3
  Constant/1 -> Product3/2, Product1/2
  [RPS] -> Square/1
  [Omega_eta] -> Cross Product2/2
  Gain/1 -> P_MY1/2
  P_MY1/1 -> Product4/2
  Cross Product2/1 -> [M_gryo]
  [T_A] -> Product4/1
  Product4/1 -> Cross Product2/1
  Constant10/1 -> P_MY1/1
  [RPS] -> Gain/1
  Add/1 -> Sum/1
  [M_gryo] -> Sum/2
  Constant6/1 -> Mux9/1
  Rotation Angles to Direction Cosine Matrix1/1 -> Transpose1/1
  Constant7/1 -> Mux9/3
  Mux9/1 -> Sum1/1
  Degrees to Radians3/1 -> Mux9/2, Tilt Prop Local Vars1/4(TiltAngle_rad)
  Degrees to Radians1/1 -> Sum1/2, Tilt Prop Local Vars1/8(PropAng_b2p_rad)
  Sum1/1 -> Rotation Angles to Direction Cosine Matrix1/1
  Product2/1 -> Reshape/1
  Reshape/1 -> [T_A]
  Transpose1/1 -> Product2/1
  Constant8/1 -> Product2/2

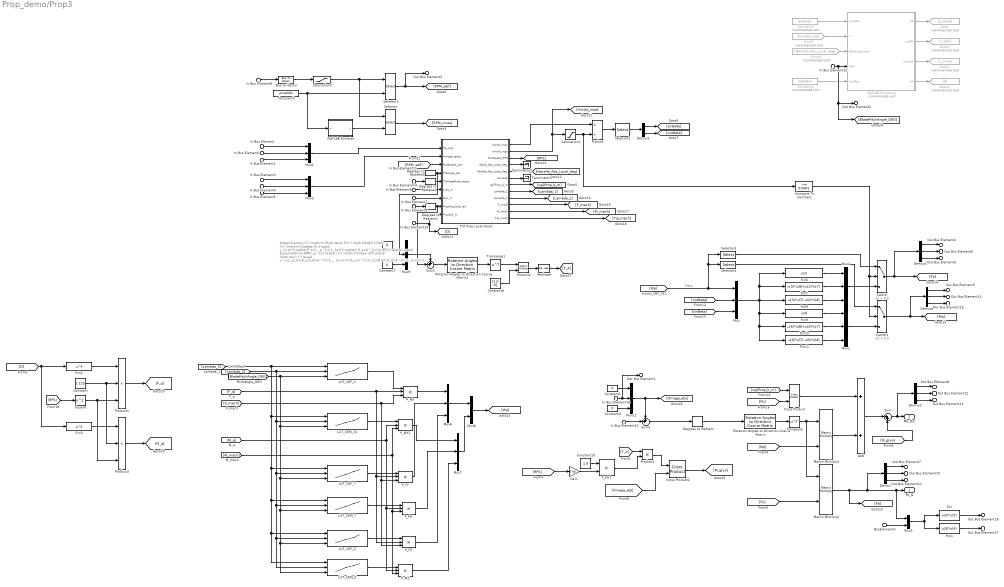
== system Prop_demo/Prop3 ==
  note: $\begin{array}{l} \mathrm{Prop\ Aero\ Fit\ /\ Coef\ Model}\\[3pt] (1)\ \mathrm{Sweep\ fit:}\quad y_{c,p}(V,\alpha,R_p)=a^{(c)}_{p}(V,\alpha)\,R_p+b^{(c)}_{p}(V,\alpha),\quad R_p=\mathrm{RPM}_p^{2}.\\[5pt] (2)\ \mathrm{Coax\ diff\ plane\ (one\ pair):}\\ \quad y^{u}_{c}(V,R_u,R_d)=k^{(c)}_{uu}(V)\,R_u+k^{(c)}_{ud}(V)\,R_d+b^{(c)}_{u}(V),\\ \quad y^{d}_{c}(V,R_u,R_d)=k^{(c)}_{du}(V)\,R_u+k^{(c)}_{dd}(V)\,R_d+b^{(c)}_{d}(V).\\[5pt] (3)\ \mathrm{Ratio\ (split\ of\ slope):}\quad s^{(c)}_{u}=k^{(c)}_{uu}+k^{(c)}_{ud},\quad s^{(c)}_{d}=k^{(c)}_{dd}+k^{(c)}_{du},\\ \quad r^{(c)}_{uu}=\frac{k^{(c)}_{uu}}{s^{(c)}_{u}},\quad r^{(c)}_{ud}=\frac{k^{(c)}_{ud}}{s^{(c)}_{u}},\quad r^{(c)}_{dd}=\frac{k^{(c)}_{dd}}{s^{(c)}_{d}},\quad r^{(c)}_{du}=\frac{k^{(c)}_{du}}{s^{(c)}_{d}}.\\[5pt] (4)\ \mathrm{Coax\ weight:}\quad s=(\cos(\alpha))^{p},\quad p=\mathrm{coaxAlphaPow}.\\ \quad \mathrm{upper:}\quad a^{(c)}_{\mathrm{self}}=s\,r^{(c)}_{uu}\,a^{(c)}_{p},\quad a^{(c)}_{\mathrm{cross}}=s\,r^{(c)}_{ud}\,a^{(c)}_{p},\\ \quad \mathrm{lower:}\quad a^{(c)}_{\mathrm{self}}=s\,r^{(c)}_{dd}\,a^{(c)}_{p},\quad a^{(c)}_{\mathrm{cross}}=s\,r^{(c)}_{du}\,a^{(c)}_{p}.\\[5pt] (5)\ \mathrm{Final\ prediction:}\quad \hat y_{c,p}=a^{(c)}_{\mathrm{self}}\,R_p+a^{(c)}_{\mathrm{cross}}\,R_{m(p)}+b^{(c)}_{p}(V,\alpha). \end{array}$
  In Bus Element6 : Inport  PortName=omegaProp_RPM
      settings: AttributesFormatString=%<OutDataTypeStr>\nDimensions: %<PortDimensions>
  In Bus Element14 : Inport  Port=2  PortName=TiltAct  Element=TiltAngleRate_dps
  In Bus Element15 : Inport  Port=2  PortName=TiltAct  Element=BladePitchAngle_DEG
  In Bus Element11 : Inport  Port=2  PortName=TiltAct  Element=TiltAngle_DEG
  In Bus Element16 : Inport  Port=2  PortName=TiltAct  Element=TiltAngle_DEG
  In Bus Element13 : Inport  Port=3  PortName=GeomProp  Element=PropAng_b2p_deg
      settings: AttributesFormatString=%<OutDataTypeStr>\nDimensions: %<PortDimensions>
  In Bus Element9 : Inport  Port=3  PortName=GeomProp  Element=PropAng_b2p_deg
      settings: AttributesFormatString=%<OutDataTypeStr>\nDimensions: %<PortDimensions>
  In Bus Element10 : Inport  Port=3  PortName=GeomProp  Element=PropDia_m
      settings: AttributesFormatString=%<OutDataTypeStr>\nDimensions: %<PortDimensions>
  In Bus Element8 : Inport  Port=3  PortName=GeomProp  Element=cg2PropHinge_b_m
      settings: AttributesFormatString=%<OutDataTypeStr>\nDimensions: %<PortDimensions>
  BusElementIn : Inport  Port=3  PortName=GeomProp  Element=cg2PropHinge_b_m
  In Bus Element7 : Inport  Port=3  PortName=GeomProp  Element=TiltArm_m
      settings: AttributesFormatString=%<OutDataTypeStr>\nDimensions: %<PortDimensions>
  In Bus Element : Inport  Port=4  PortName=EOM  Element=VB_mps.Ub_mps
      settings: AttributesFormatString=%<OutDataTypeStr>\nDimensions: %<PortDimensions>
  In Bus Element1 : Inport  Port=4  PortName=EOM  Element=VB_mps.Vb_mps
      settings: AttributesFormatString=%<OutDataTypeStr>\nDimensions: %<PortDimensions>
  In Bus Element2 : Inport  Port=4  PortName=EOM  Element=VB_mps.Wb_mps
      settings: AttributesFormatString=%<OutDataTypeStr>\nDimensions: %<PortDimensions>
  In Bus Element3 : Inport  Port=4  PortName=EOM  Element=Rates_radps.P_radps
      settings: AttributesFormatString=%<OutDataTypeStr>\nDimensions: %<PortDimensions>
  In Bus Element4 : Inport  Port=4  PortName=EOM  Element=Rates_radps.Q_radps
      settings: AttributesFormatString=%<OutDataTypeStr>\nDimensions: %<PortDimensions>
  In Bus Element5 : Inport  Port=4  PortName=EOM  Element=Rates_radps.R_radps
      settings: AttributesFormatString=%<OutDataTypeStr>\nDimensions: %<PortDimensions>
  Add : Sum
  Bus to Vector : BusToVector
  Compare To Constant : simulink/Logic and Bit Operations/Compare To Constant  relop=<=  const=0.0001  OutDataTypeStr=boolean
  Constant : Constant  Value=1.225
  Constant{1..2,6..7} (4 alike) : Constant  Value=0
  Constant10 : Constant  Value=1.0
  Constant3 : Constant  Value=propAbs
  Constant4 : Constant  Commented=on  Value=CoefBus  OutDataTypeStr=Bus: CoefBusObj
  Constant5 : Constant  Commented=on  Value=propAbs
  Constant8 : Constant  Value=[1 0 0]
  Cross Product : matrix_library/Cross Product
  Cross Product2 : matrix_library/Cross Product
  Degrees to Radians{,1..3} (4 alike) : simulink_extras/Transformations/Degrees to Radians
  Demux{,2..4} (4 alike) : Demux  Outputs=3
  Demux1 : Demux  Outputs=2
  Fcn : Fcn  Expr=u(3)*u(5)
  Fcn1 : Fcn  Expr=u(3)*u(4)
  Fcn10 : Fcn  Expr=u(6)*u(8)+u(5)*u(7)
  Fcn11 : Fcn  Expr=u(6)*u(7)-u(5)*u(8)
  Fcn2 : Fcn  Expr=u^4
  Fcn3 : Fcn  Expr=u^5
  Fcn6 : Fcn  Expr=u(1)
  Fcn7 : Fcn  Expr=u(3)*u(8)+u(2)*u(7)
  Fcn8 : Fcn  Expr=u(3)*u(7)-u(2)*u(8)
  Fcn9 : Fcn  Expr=u(4)
  From6 : From  Commented=on  GotoTag=Nacelle_Abs_Local_deg
  From7 : From  Commented=on  GotoTag=Vmold_mps
  Gain : Gain  Gain=2*pi
  Goto : Goto  Commented=on  GotoTag=a_base
  Goto1 : Goto  Commented=on  GotoTag=r_self
  Goto2 : Goto  Commented=on  GotoTag=r_cross
  Goto3 : Goto  Commented=on  GotoTag=b
  LUT_CEF_X : Lookup_n-D  NumberOfTableDimensions=3  BreakpointsForDimension1=cfd3d_ja  BreakpointsForDimension2=cfd3d_jl  BreakpointsForDimension3=cfd3d_pitch  Table=cfd3d_P2_CEF_X  ExtrapMethod=Clip  UseLastTableValue=on  InternalRulePriority=Speed  RndMeth=Simplest
      settings: InputPortMap=u0,u1,u2
  LUT_CEF_Y : Lookup_n-D  NumberOfTableDimensions=3  BreakpointsForDimension1=cfd3d_ja  BreakpointsForDimension2=cfd3d_jl  BreakpointsForDimension3=cfd3d_pitch  Table=cfd3d_P2_CEF_Y  ExtrapMethod=Clip  UseLastTableValue=on  InternalRulePriority=Speed  RndMeth=Simplest
      settings: InputPortMap=u0,u1,u2
  LUT_CEF_Z : Lookup_n-D  NumberOfTableDimensions=3  BreakpointsForDimension1=cfd3d_ja  BreakpointsForDimension2=cfd3d_jl  BreakpointsForDimension3=cfd3d_pitch  Table=cfd3d_P2_CEF_Z  ExtrapMethod=Clip  UseLastTableValue=on  InternalRulePriority=Speed  RndMeth=Simplest
      settings: InputPortMap=u0,u1,u2
  LUT_CEM_X1 : Lookup_n-D  NumberOfTableDimensions=3  BreakpointsForDimension1=cfd3d_ja  BreakpointsForDimension2=cfd3d_jl  BreakpointsForDimension3=cfd3d_pitch  Table=cfd3d_P2_CEM_X  ExtrapMethod=Clip  UseLastTableValue=on  InternalRulePriority=Speed  RndMeth=Simplest
      settings: InputPortMap=u0,u1,u2
  LUT_CEM_Y : Lookup_n-D  NumberOfTableDimensions=3  BreakpointsForDimension1=cfd3d_ja  BreakpointsForDimension2=cfd3d_jl  BreakpointsForDimension3=cfd3d_pitch  Table=cfd3d_P2_CEM_Y  ExtrapMethod=Clip  UseLastTableValue=on  InternalRulePriority=Speed  RndMeth=Simplest
      settings: InputPortMap=u0,u1,u2
  LUT_CEM_Z : Lookup_n-D  NumberOfTableDimensions=3  BreakpointsForDimension1=cfd3d_ja  BreakpointsForDimension2=cfd3d_jl  BreakpointsForDimension3=cfd3d_pitch  Table=cfd3d_P2_CEM_Z  ExtrapMethod=Clip  UseLastTableValue=on  InternalRulePriority=Speed  RndMeth=Simplest
      settings: InputPortMap=u0,u1,u2
  MATLAB Function : MATLAB Function  TreatAsAtomicUnit=on
  MATLAB Function2 : MATLAB Function  Commented=on  TreatAsAtomicUnit=on
  Matrix Multiply1 : Product  Multiplication=Matrix(*)
  Matrix Multiply2 : Product  Multiplication=Matrix(*)
  Mux{,1..4,6..7,9,11} (9 alike) : Mux  Inputs=3
  Mux5 : Mux  Inputs=2
  Mux8 : Mux  Inputs=2
  P_FY : Product  Inputs=***
  P_FZ : Product  Inputs=***
  P_MX : Product  Inputs=***
  P_MX1 : Product  Inputs=***
  P_MY : Product  Inputs=***
  P_MY1 : Product  Inputs=**
  P_MZ : Product  Inputs=***
  Product : Product  Inputs=*/
  Product1 : Product  Inputs=3
  Product2 : Product  Multiplication=Matrix(*)
  Product3 : Product  Inputs=3
  Product4 : Product
  Reshape : Reshape
  Rotation Angles to Direction Cosine Matrix : sharedtransform/Rotation Angles to Direction Cosine Matrix  rotationOrder=XYZ  aMode=aMode
  Rotation Angles to Direction Cosine Matrix1 : sharedtransform/Rotation Angles to Direction Cosine Matrix  rotationOrder=XYZ  aMode=aMode
  Saturation1 : Saturate  UpperLimit=inf  LowerLimit=0.0001
  Saturation2 : Saturate  UpperLimit=1500  LowerLimit=0
      settings: AttributesFormatString=min: %<LowerLimit>\nmax: %<UpperLimit>
  Selector : Selector  InputPortWidth=8  IndexOptions=Index vector (port)  Indices=[1 3]  OutputSizes=1
  Selector1 : Selector  InputPortWidth=8  IndexOptions=Index vector (port)  Indices=[1 3]  OutputSizes=1
  Selector2 : Selector  InputPortWidth=3  IndexOptions=Index vector (dialog)  Indices=[2 3]  OutputSizes=1
  Selector3 : Selector  InputPortWidth=6  IndexOptions=Index vector (dialog)  Indices=[1 2 3]  OutputSizes=1
  Selector4 : Selector  InputPortWidth=6  IndexOptions=Index vector (dialog)  Indices=[4 5 6]  OutputSizes=1
  Square : Math  Operator=square
  Sum : Sum  Inputs=|++
  Sum1 : Sum  Inputs=++|
  Sum5 : Sum  Inputs=++|
  Switch : Switch  Criteria=u2 > Threshold  Threshold=0.5  SaturateOnIntegerOverflow=off  InputSameDT=off
  Switch1 : Switch  Criteria=u2 > Threshold  Threshold=0.5  SaturateOnIntegerOverflow=off  InputSameDT=off
  Terminator1 : Terminator
  Terminator2 : Terminator
  Tilt Prop Local Vars1 : Subsystem  AncestorBlock=DF3000_V2_Common/Tilt Prop Local Vars1
  Transpose : Math  Operator=transpose
  Transpose1 : Math  Operator=transpose
  Fb_N : Outport  PortDimensions=3
  Mb_Nm : Outport  Port=2  PortDimensions=3
  Out Bus Element7 : Outport  Port=3  PortName=Data  Element=Fx_Prop
  Out Bus Element10 : Outport  Port=3  PortName=Data  Element=Fy_Prop
  Out Bus Element11 : Outport  Port=3  PortName=Data  Element=Fz_Prop
  Out Bus Element8 : Outport  Port=3  PortName=Data  Element=Mx_Prop
  Out Bus Element12 : Outport  Port=3  PortName=Data  Element=My_Prop
  Out Bus Element13 : Outport  Port=3  PortName=Data  Element=Mz_Prop
  Out Bus Element1 : Outport  Port=3  PortName=Data  Element=TiltAngle_DEG
  Out Bus Element2 : Outport  Port=3  PortName=Data  Element=BladePitchAngle_DEG
  Out Bus Element3 : Outport  Port=3  PortName=Data  Element=RPM
  Out Bus Element4 : Outport  Port=3  PortName=Data  Element=Fx_Local
  Out Bus Element5 : Outport  Port=3  PortName=Data  Element=Fy_Local
  Out Bus Element6 : Outport  Port=3  PortName=Data  Element=Fz_Local
  Out Bus Element9 : Outport  Port=3  PortName=Data  Element=Mx_Local
  Out Bus Element14 : Outport  Port=3  PortName=Data  Element=My_Local
  Out Bus Element15 : Outport  Port=3  PortName=Data  Element=Mz_Local
  Out Bus Element16 : Outport  Port=3  PortName=Data  Element=BMbx_Prop
  Out Bus Element17 : Outport  Port=3  PortName=Data  Element=BMby_Prop
  wires:
  [RPS] -> Gain/1
  Constant10/1 -> P_MY1/1
  Product4/1 -> Cross Product2/1
  [T_A] -> Product4/1
  Cross Product2/1 -> [M_gryo]
  P_MY1/1 -> Product4/2
  Gain/1 -> P_MY1/2
  [Omega_eta] -> Cross Product2/2
  [RPS] -> Square/1
  Constant/1 -> Product1/2, Product3/2
  Square/1 -> Product1/3, Product3/3
  Product3/1 -> [M_q]
  Product1/1 -> [F_q]
  Fcn3/1 -> Product3/1
  [D] -> Fcn2/1, Fcn3/1
  Fcn2/1 -> Product1/1
  P_MX1/1 -> Mux7/1
  P_FZ/1 -> Mux6/3
  Mux8/1 -> [Wp]
  Mux7/1 -> Mux8/2
  Mux6/1 -> Mux8/1
  P_FY/1 -> Mux6/2
  P_MZ/1 -> Mux7/3
  P_MY/1 -> Mux7/2
  P_MX/1 -> Mux6/1
  LUT_CEF_X/1 -> P_MX/1
  LUT_CEF_Z/1 -> P_FZ/1
  [BladePitchAngle_DEG] -> LUT_CEF_X/3, LUT_CEM_X1/3, LUT_CEF_Y/3, LUT_CEM_Y/3, LUT_CEF_Z/3, LUT_CEM_Z/3
  [Lambda_1] -> LUT_CEM_X1/1, LUT_CEF_Y/1, LUT_CEM_Y/1, LUT_CEF_Z/1, LUT_CEM_Z/1, LUT_CEF_X/1
  [Lambda_2] -> LUT_CEF_X/2, LUT_CEM_X1/2, LUT_CEF_Y/2, LUT_CEM_Y/2, LUT_CEF_Z/2, LUT_CEM_Z/2
  [M_q] -> P_MX1/2, P_MY/2, P_MZ/2
  LUT_CEM_X1/1 -> P_MX1/1
  LUT_CEM_Y/1 -> P_MY/1
  LUT_CEM_Z/1 -> P_MZ/1
  [F_mach] -> P_FY/3, P_FZ/3, P_MX/3
  LUT_CEF_Y/1 -> P_FY/1
  [M_mach] -> P_MY/3, P_MZ/3, P_MX1/3
  [F_q] -> P_FY/2, P_FZ/2, P_MX/2
  Tilt Prop Local Vars1/12(Tip_mach) -> [Tip_mach]
  Tilt Prop Local Vars1/11(M_mach) -> [M_mach]
  Tilt Prop Local Vars1/10(F_mach) -> [F_mach]
  Tilt Prop Local Vars1/9(Lambda_2) -> [Lambda_2]
  Tilt Prop Local Vars1/8(Lambda_1) -> [Lambda_1]
  In Bus Element15/1 -> Out Bus Element2/1, [BladePitchAngle_DEG], MATLAB Function2/4(Pitch)
  In Bus Element11/1 -> Degrees to Radians3/1
  In Bus Element14/1 -> Degrees to Radians2/1
  Degrees to Radians2/1 -> Tilt Prop Local Vars1/5(TiltAngleRate_radps)
  In Bus Element7/1 -> Tilt Prop Local Vars1/7(Arm_m)
  Selector/1 -> [RPM_cross]
  MATLAB Function/1(y) -> Selector/2
  Constant3/1 -> Selector1/2, MATLAB Function/1(u)
  In Bus Element6/1 -> Bus to Vector/1
  Bus to Vector/1 -> Saturation2/1
  Saturation2/1 -> Selector/1, Selector1/1
  MATLAB Function2/1(a6) -> Goto/1
  Rotation Angles to Direction Cosine Matrix/1 -> Transpose/1
  [cg2Prop_b_m] -> Cross Product/1
  Cross Product/1 -> Add/1
  Sum5/1 -> Degrees to Radians/1
  Degrees to Radians/1 -> Rotation Angles to Direction Cosine Matrix/1
  Matrix Multiply1/1 -> Add/2
  [Mp] -> Matrix Multiply1/2
  Transpose/1 -> Matrix Multiply2/1, Matrix Multiply1/1
  Selector1/1 -> Out Bus Element3/1, [RPM_self]
  In Bus Element8/1 -> Tilt Prop Local Vars1/6(Lvec_m)
  In Bus Element9/1 -> Degrees to Radians1/1
  In Bus Element/1 -> Mux2/1
  In Bus Element5/1 -> Mux3/3
  In Bus Element4/1 -> Mux3/2
  In Bus Element3/1 -> Mux3/1
  In Bus Element2/1 -> Mux2/3
  In Bus Element10/1 -> Tilt Prop Local Vars1/9(PropDia_m), [D]
  Mux3/1 -> Tilt Prop Local Vars1/2(omega_radps)
  Mux2/1 -> Tilt Prop Local Vars1/1(Vb_mps)
  In Bus Element1/1 -> Mux2/2
  [RPM_self] -> Tilt Prop Local Vars1/3(RotSpeed_rpm)
  Tilt Prop Local Vars1/1(VLocal_mps) -> Product/1
  Tilt Prop Local Vars1/2(Vmold_mps) -> Saturation1/1, [Vmold_mps]
  Product/1 -> Selector2/1
  Selector2/1 -> Demux1/1
  Tilt Prop Local Vars1/3(RotSpeed_RPS) -> [RPS]
  Tilt Prop Local Vars1/6(Lambda) -> Terminator1/1
  Constant4/1 -> MATLAB Function2/5(CoefBus)
  Constant5/1 -> MATLAB Function2/1(propAbs)
  MATLAB Function2/4(b6) -> Goto3/1
  MATLAB Function2/3(r_cross6) -> Goto2/1
  MATLAB Function2/2(r_self6) -> Goto1/1
  From6/1 -> MATLAB Function2/3(Alpha_abs_local)
  From7/1 -> MATLAB Function2/2(V)
  [cosBeta] -> Mux/2
  [sinBeta] -> Mux/3
  Mux/1 -> Fcn8/1, Fcn7/1, Fcn6/1, Fcn9/1, Fcn11/1, Fcn10/1
  Fcn9/1 -> Mux1/1
  Fcn10/1 -> Mux1/2
  Fcn11/1 -> Mux1/3
  Mux1/1 -> Switch1/3
  Fcn6/1 -> Mux4/1
  Fcn7/1 -> Mux4/2
  Fcn8/1 -> Mux4/3
  Mux4/1 -> Switch/3
  [Fp] -> Matrix Multiply2/2
  [Fb] -> Cross Product/2
  [Wp] -> Selector4/1, Selector3/1, Mux/1  "FMpw"
  Demux/1 -> Out Bus Element7/1
  Demux/2 -> Out Bus Element10/1
  Demux/3 -> Out Bus Element11/1
  Demux2/3 -> Out Bus Element13/1
  Demux2/2 -> Out Bus Element12/1
  Demux2/1 -> Out Bus Element8/1
  Mux11/1 -> Sum5/1, [Omega_eta]
  Constant2/1 -> Mux11/3
  Constant1/1 -> Mux11/1
  In Bus Element16/1 -> Out Bus Element1/1, Mux11/2
  In Bus Element13/1 -> Sum5/2
  Demux1/1 -> [sinBeta]
  Demux1/2 -> [cosBeta]
  Tilt Prop Local Vars1/4(Alpha_Abs_Local_deg) -> Terminator2/1
  Tilt Prop Local Vars1/5(Nacelle_Abs_Local_deg) -> [Nacelle_Abs_Local_deg]
  Tilt Prop Local Vars1/7(cg2Prop_b_m) -> [cg2Prop_b_m]
  Saturation1/1 -> Compare To Constant/1, Product/2
  Selector3/1 -> Switch/1
  Selector4/1 -> Switch1/1
  Compare To Constant/1 -> Switch1/2, Switch/2
  Switch/1 -> Demux3/1, [Fp]
  Demux3/3 -> Out Bus Element6/1
  Demux3/1 -> Out Bus Element4/1
  Demux3/2 -> Out Bus Element5/1
  Demux4/3 -> Out Bus Element15/1
  Switch1/1 -> [Mp], Demux4/1
  Demux4/1 -> Out Bus Element9/1
  Demux4/2 -> Out Bus Element14/1
  Matrix Multiply2/1 -> Demux/1, Mux5/1, Fb_N/1, [Fb]
  Fcn/1 -> Out Bus Element16/1
  Mux5/1 -> Fcn1/1, Fcn/1
  BusElementIn/1 -> Mux5/2
  Fcn1/1 -> Out Bus Element17/1
  [M_gryo] -> Sum/2
  Sum/1 -> Demux2/1, Mb_Nm/1
  Add/1 -> Sum/1
  Transpose1/1 -> Product2/1
  Constant8/1 -> Product2/2
  Degrees to Radians1/1 -> Sum1/2, Tilt Prop Local Vars1/8(PropAng_b2p_rad)
  Degrees to Radians3/1 -> Mux9/2, Tilt Prop Local Vars1/4(TiltAngle_rad)
  Constant7/1 -> Mux9/3
  Reshape/1 -> [T_A]
  Rotation Angles to Direction Cosine Matrix1/1 -> Transpose1/1
  Mux9/1 -> Sum1/1
  Sum1/1 -> Rotation Angles to Direction Cosine Matrix1/1
  Product2/1 -> Reshape/1
